simulink model "S_FUNC_ADD_SUB"  (R2018b)
settings: Solver=VariableStepAuto  StartTime=0.0  StopTime=10.0  RelTol=1e-3
settings Model: Creator=student  LastModifiedBy=student

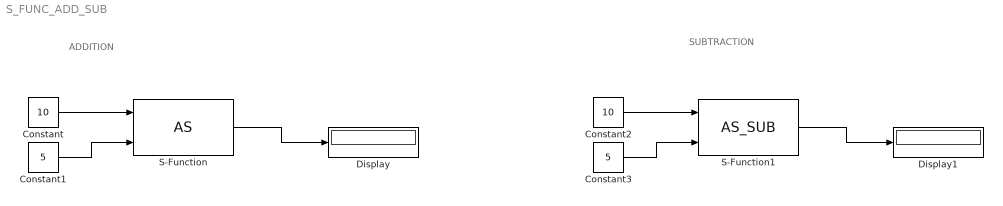
== system S_FUNC_ADD_SUB ==
  note: SUBTRACTION
  note: ADDITION
  Constant : Constant  Value=10
  Constant1 : Constant  Value=5
  Constant2 : Constant  Value=10
  Constant3 : Constant  Value=5
  Display : Display
  Display1 : Display
  S-Function : S-Function  FunctionName=AS  SFunctionDeploymentMode=off  EnableBusSupport=off
  S-Function1 : S-Function  FunctionName=AS_SUB  SFunctionDeploymentMode=off  EnableBusSupport=off
  wires:
  Constant/1 -> S-Function/1
  Constant1/1 -> S-Function/2
  S-Function/1 -> Display/1
  S-Function1/1 -> Display1/1
  Constant3/1 -> S-Function1/2
  Constant2/1 -> S-Function1/1
